simulink model "model_2022b1"  (R2022b)
settings: Solver=FixedStepAuto  StartTime=0.0  StopTime=20  FixedStep=0.001  RelTol=1e-3
undefined symbols (not defined in the file or in its folder): A, A0f, b, d, gamma, N, P
settings Model: Creator=Катя  LastModifiedBy=R1505-We2-6-Stud
settings OptimizationCC: ReuseModelBlockBuffer=on

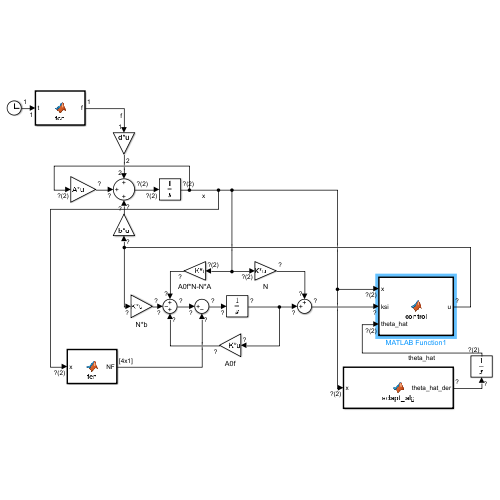
[thumbnail: Simulink's stored preview of the top-level diagram]
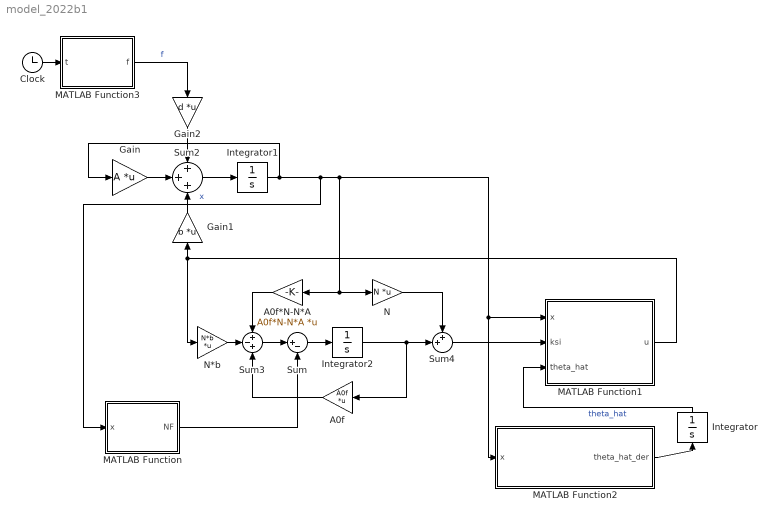
== system model_2022b1 ==
  A0f : Gain  Gain=A0f  Multiplication=Matrix(K*u)
  A0f*N-N*A : Gain  Gain=A0f*N-N*A  Multiplication=Matrix(K*u)
  Clock : Clock
  Gain : Gain  Gain=A  Multiplication=Matrix(K*u)
  Gain1 : Gain  Gain=b  Multiplication=Matrix(K*u)
  Gain2 : Gain  Gain=d  Multiplication=Matrix(K*u)
  Integrator : Integrator  InitialCondition=[0;0]
  Integrator1 : Integrator
  Integrator2 : Integrator
  MATLAB Function : MATLAB Function  TreatAsAtomicUnit=on
  MATLAB Function1 : MATLAB Function  TreatAsAtomicUnit=on
  MATLAB Function2 : MATLAB Function  TreatAsAtomicUnit=on
  MATLAB Function3 : MATLAB Function  TreatAsAtomicUnit=on
  N : Gain  Gain=N  Multiplication=Matrix(K*u)
  N*b : Gain  Gain=N*b  Multiplication=Matrix(K*u)
  Sum : Sum  Inputs=|+-
  Sum2 : Sum  Inputs=+++
  Sum3 : Sum  Inputs=+-+
  Sum4 : Sum  Inputs=++|
  wires:
  Integrator1/1 -> MATLAB Function/1(x), MATLAB Function2/1(x), MATLAB Function1/1(x), N/1, A0f*N-N*A/1, Gain/1  "x"
  MATLAB Function2/1(theta_hat_der) -> Integrator/1
  Integrator/1 -> MATLAB Function1/3(theta_hat)  "theta_hat"
  Gain/1 -> Sum2/2
  Gain1/1 -> Sum2/3
  Sum2/1 -> Integrator1/1
  Gain2/1 -> Sum2/1
  MATLAB Function3/1(f) -> Gain2/1  "f"
  Integrator2/1 -> A0f/1, Sum4/2
  Sum3/1 -> Sum/1
  A0f/1 -> Sum3/3
  N*b/1 -> Sum3/2
  A0f*N-N*A/1 -> Sum3/1
  MATLAB Function1/1(u) -> N*b/1, Gain1/1
  N/1 -> Sum4/1
  Sum4/1 -> MATLAB Function1/2(ksi)
  Sum/1 -> Integrator2/1
  MATLAB Function/1(NF) -> Sum/2
  Clock/1 -> MATLAB Function3/1(t)

== matlab function model_2022b1/MATLAB Function1 ==
  data: x input size=2; u output size=1; ksi input; theta_hat input; K parameter
function u = control(x, ksi, theta_hat, K)
    u = -K*x-theta_hat.'*ksi-11*sin(x(2)^2-3*x(1));
end

== matlab function model_2022b1/MATLAB Function ==
  data: x input; NF output; N parameter
function NF = fcn(x, N)

NF = N*[0; 11*sin(x(2)^2-3*x(1))];

== matlab function model_2022b1/MATLAB Function2 ==
  data: x input; theta_hat_der output; gamma parameter; b parameter; P parameter
function theta_hat_der = adapt_alg(x, gamma, b, P)
    theta_hat_der = gamma * ksi * b.' * P * x;
end

== matlab function model_2022b1/MATLAB Function3 ==
  data: t input; f output; th parameter
function f = fcn(t, th)

f = cos(th^2*t)*cos(th*t);
